simulink model "OffsetRemover"  (R2023a)
settings: Solver=FixedStepAuto  StartTime=0.0  StopTime=100  FixedStep=0.0001  RelTol=1e-3
libraries: dspstat3 x1
settings Model: Creator=JesseJabezArendse  LastModifiedBy=JesseJabezArendse
settings DebuggingCC: UnderSpecifiedDimensionMsg=warning

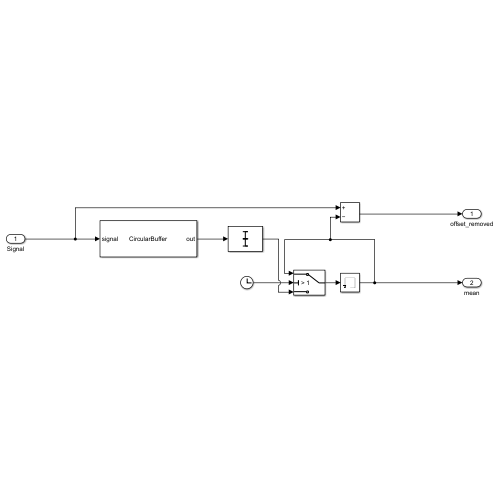
[thumbnail: Simulink's stored preview of the top-level diagram]
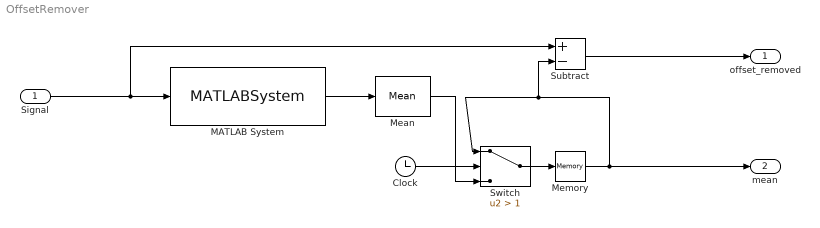
== system OffsetRemover ==
  Signal : Inport  PortDimensions=1  Interpolate=off
  Clock : Clock
  MATLAB System : MATLABSystem  System=CircularBuffer  BufferLength=circularBufferSize  InitialCondition=0  SimulateUsing=Code generation
      mask Type: CircularBuffer
      mask Display:
      | disp('CircularBuffer');
      | port_label('input',1,'signal');
      | port_label('output',1,'out');
  Mean : dspstat3/Mean  run=off  InputProcessing=Columns as channels (frame based)  reset_popup=None  directionMode=Entire input  dimension=1  roiEnable=off  roiType=Rectangles  roiPortion=Entire ROI  roiOutput=Individual statistics for each ROI  roiFlag=off  roundingMode=Floor  overflowMode=off  outputDataTypeStr=Inherit: Same as accumulator  outputMin=[]  outputMax=[]  outputLastDataTypeStr=Inherit: Same as accumulator
  Memory : Memory
  Subtract : Sum  Inputs=+-
  Switch : Switch  Criteria=u2 > Threshold  Threshold=1  SaturateOnIntegerOverflow=off  InputSameDT=off
  offset_removed : Outport
  mean : Outport  Port=2
  wires:
  Signal/1 -> Subtract/1, MATLAB System/1
  MATLAB System/1 -> Mean/1
  Mean/1 -> Switch/3
  Clock/1 -> Switch/2
  Switch/1 -> Memory/1
  Memory/1 -> mean/1, Switch/1, Subtract/2
  Subtract/1 -> offset_removed/1
